simulink model "DIG_IF_test"  (R2021b)
settings: Solver=FixedStepDiscrete  StartTime=0.0  StopTime=stop_time-1  RelTol=1e-3
undefined symbols (not defined in the file): input_bus
libraries: dspsrcs4 x22
settings Model: DataTypeOverride=Off  Creator=torha  LastModifiedBy=torha
settings SolverCC: AlgebraicLoopSolver=TrustRegion
settings OptimizationCC: BlockReduction=off  ConditionallyExecuteInputs=off  DefaultParameterBehavior=Inlined  InheritOutputTypeSmallerThanSingle=on
settings DebuggingCC: AlgebraicLoopMsg=error  SingleTaskRateTransMsg=error  SFMachineParentedDataDiag=warning
settings HardwareCC: ProdBitPerPointer=32  ProdBitPerSizeT=32  ProdBitPerPtrDiffT=32  ProdLargestAtomicFloat=None  ProdIntDivRoundTo=Undefined  ProdEndianess=Unspecified  ProdWordSize=32  ProdHWDeviceType=ASIC/FPGA->ASIC/FPGA  TargetBitPerPointer=64  TargetBitPerSizeT=64  TargetBitPerPtrDiffT=64  TargetLongLongMode=on  TargetIntDivRoundTo=Zero  TargetEndianess=LittleEndian  TargetWordSize=64  TargetHWDeviceType=Custom Processor->MATLAB Host Computer  ProdEqTarget=off

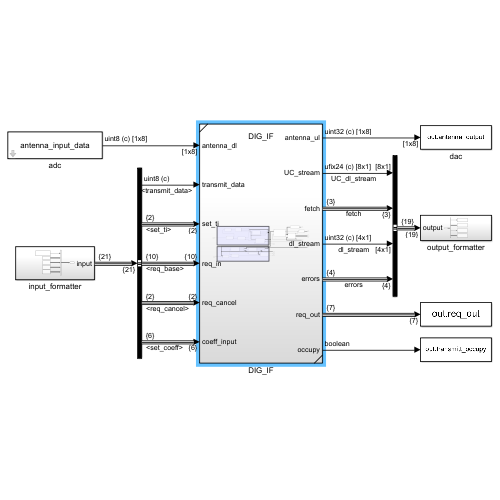
[thumbnail: Simulink's stored preview of the top-level diagram]
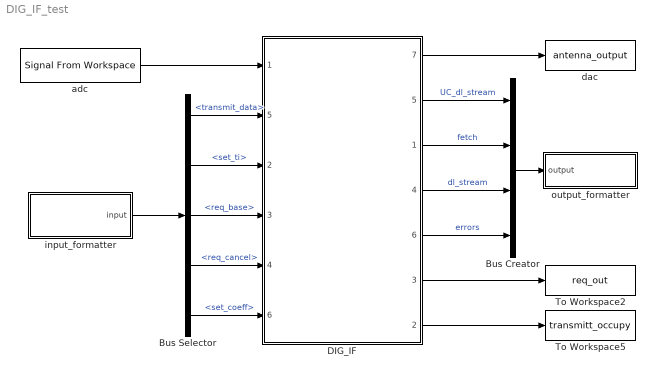
== system DIG_IF_test ==
  Bus Creator : BusCreator  Inputs=4
  Bus Selector : BusSelector  OutputSignals=transmit_data,set_ti,req_base,req_cancel,set_coeff
  DIG_IF : Subsystem  ReferencedSubsystem=DIG_IF
      settings: PortSchema="{\"entries\":[{\"content\":{\"sides\":[{\"content\":{\"connectorIds\":[\"Out7\",\"Out5\",\"Out1\",\"Out4\",\"Out6\",\"Out3\",\"Out2\"]},\"type\":\"ConnectorPlacement.EquallySpacedRectSide\",\"uuid\":\"0a36bb2c-b508-4463-a150-0627b474e72d\"},{\"content\":{\"connectorIds\":[\"In1\",\"In5\",\"In2\",\"In3\",\"In4\",\"In6\"],\"side\":\"RIGHT\"},\"type\":\"ConnectorPlacement.EquallySpacedRectSide\",\"uuid\":\"4cc461b4-d2d5-47e9-bf85-abb0cb83a1e3\"},{\"content\":{\"connectorIds\":[],\"side\":\"TOP\"},\"type\":\"ConnectorPlacement.EquallySpacedRectSide\",\"uuid\":\"3f3acd78-cd76-4a3f-93f8-4cd9f7c1daae\"},{\"content\":{\"connectorIds\":[],\"side\":\"BOTTOM\"},\"type\":\"ConnectorPlacement.EquallySpacedRectSide\",\"uuid\":\"e0439bc9-96cc-469d-b0c1-4082506a186c\"}]},\"type\":\"ConnectorPlacement.EquallySpacedConnector\",\"uuid\":\"66db1979-25ee-4b63-8861-56a9b0aa4b63\"}],\"packageUris\":[\"http://schema.mathworks.com/mf0/Connector/R2020b\"],\"version\":\"1.0\"}"
  To Workspace2 : ToWorkspace  VariableName=req_out  SaveFormat=Timeseries  SampleTime=-1
      settings: Save2DSignal=2-D array (concatenate along first dimension)
  To Workspace5 : ToWorkspace  VariableName=transmitt_occupy  SampleTime=-1
      settings: Save2DSignal=2-D array (concatenate along first dimension)
  adc : dspsrcs4/Signal From Workspace  X=antenna_input_data  Ts=1  nsamps=1  OutputAfterFinalValue=Setting to zero  ignoreOrWarnInputAndFrameLengths=off  OutputFrames=off
  dac : ToWorkspace  VariableName=antenna_output  SaveFormat=Timeseries  SampleTime=-1
  input_formatter : Subsystem
  output_formatter : Subsystem
  wires:
  Bus Selector/1 -> DIG_IF/5  "<transmit_data>"
  adc/1 -> DIG_IF/1
  DIG_IF/7 -> dac/1
  DIG_IF/2 -> To Workspace5/1
  DIG_IF/3 -> To Workspace2/1
  Bus Selector/3 -> DIG_IF/3  "<req_base>"
  Bus Selector/5 -> DIG_IF/6  "<set_coeff>"
  Bus Selector/2 -> DIG_IF/2  "<set_ti>"
  Bus Selector/4 -> DIG_IF/4  "<req_cancel>"
  input_formatter/1(input) -> Bus Selector/1
  DIG_IF/5 -> Bus Creator/1  "UC_dl_stream"
  DIG_IF/1 -> Bus Creator/2  "fetch"
  DIG_IF/4 -> Bus Creator/3  "dl_stream"
  DIG_IF/6 -> Bus Creator/4  "errors"
  Bus Creator/1 -> output_formatter/1(output)

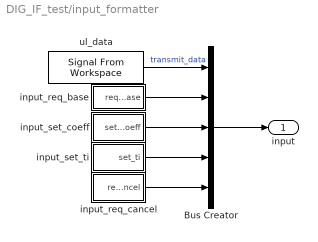
== system DIG_IF_test/input_formatter ==
  Bus Creator : BusCreator  Inputs=5
  input_req_base : Subsystem
  input_req_cancel : Subsystem
  input_set_coeff : Subsystem
  input_set_ti : Subsystem
  ul_data : dspsrcs4/Signal From Workspace  X=input_transmit_data  Ts=1  nsamps=1  OutputAfterFinalValue=Setting to zero  ignoreOrWarnInputAndFrameLengths=off  OutputFrames=off
  input : Outport
  wires:
  input_req_cancel/1(req_cancel) -> Bus Creator/5
  input_set_ti/1(set_ti) -> Bus Creator/4
  input_set_coeff/1(set_coeff) -> Bus Creator/3
  input_req_base/1(req_base) -> Bus Creator/2
  Bus Creator/1 -> input/1
  ul_data/1 -> Bus Creator/1  "transmit_data"

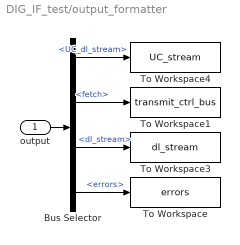
== system DIG_IF_test/output_formatter ==
  output : Inport
  Bus Selector : BusSelector  OutputSignals=UC_dl_stream,fetch,dl_stream,errors
  To Workspace : ToWorkspace  VariableName=errors  SaveFormat=Timeseries  SampleTime=-1
  To Workspace1 : ToWorkspace  VariableName=transmit_ctrl_bus  SaveFormat=Timeseries  SampleTime=-1
  To Workspace3 : ToWorkspace  VariableName=dl_stream  SampleTime=-1
      settings: Save2DSignal=2-D array (concatenate along first dimension)
  To Workspace4 : ToWorkspace  VariableName=UC_stream  SampleTime=-1
      settings: Save2DSignal=2-D array (concatenate along first dimension)
  wires:
  Bus Selector/3 -> To Workspace3/1  "<dl_stream>"
  Bus Selector/4 -> To Workspace/1  "<errors>"
  Bus Selector/1 -> To Workspace4/1  "<UC_dl_stream>"
  Bus Selector/2 -> To Workspace1/1  "<fetch>"
  output/1 -> Bus Selector/1

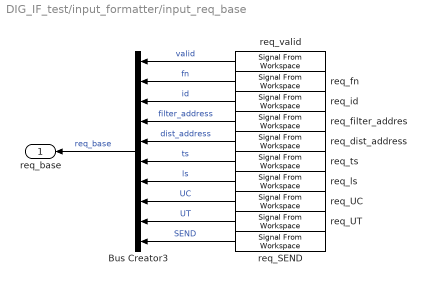
== system DIG_IF_test/input_formatter/input_req_base ==
  Bus Creator3 : BusCreator  Inputs=10
  req_SEND : dspsrcs4/Signal From Workspace  X=[horzcat([input_bus.req_base]).SEND].'  Ts=1  nsamps=1  OutputAfterFinalValue=Setting to zero  ignoreOrWarnInputAndFrameLengths=off  OutputFrames=off
  req_UC : dspsrcs4/Signal From Workspace  X=[horzcat([input_bus.req_base]).UC].'  Ts=1  nsamps=1  OutputAfterFinalValue=Setting to zero  ignoreOrWarnInputAndFrameLengths=off  OutputFrames=off
  req_UT : dspsrcs4/Signal From Workspace  X=[horzcat([input_bus.req_base]).UT].'  Ts=1  nsamps=1  OutputAfterFinalValue=Setting to zero  ignoreOrWarnInputAndFrameLengths=off  OutputFrames=off
  req_dist_address : dspsrcs4/Signal From Workspace  X=[horzcat([input_bus.req_base]).dist_address].'  Ts=1  nsamps=1  OutputAfterFinalValue=Setting to zero  ignoreOrWarnInputAndFrameLengths=off  OutputFrames=off
  req_filter_addres : dspsrcs4/Signal From Workspace  X=[horzcat([input_bus.req_base]).filter_address].'  Ts=1  nsamps=1  OutputAfterFinalValue=Setting to zero  ignoreOrWarnInputAndFrameLengths=off  OutputFrames=off
  req_fn : dspsrcs4/Signal From Workspace  X=[horzcat([input_bus.req_base]).fn].'  Ts=1  nsamps=1  OutputAfterFinalValue=Setting to zero  ignoreOrWarnInputAndFrameLengths=off  OutputFrames=off
  req_id : dspsrcs4/Signal From Workspace  X=[horzcat([input_bus.req_base]).id].'  Ts=1  nsamps=1  OutputAfterFinalValue=Setting to zero  ignoreOrWarnInputAndFrameLengths=off  OutputFrames=off
  req_ls : dspsrcs4/Signal From Workspace  X=[horzcat([input_bus.req_base]).ls].'  Ts=1  nsamps=1  OutputAfterFinalValue=Setting to zero  ignoreOrWarnInputAndFrameLengths=off  OutputFrames=off
  req_ts : dspsrcs4/Signal From Workspace  X=[horzcat([input_bus.req_base]).ts].'  Ts=1  nsamps=1  OutputAfterFinalValue=Setting to zero  ignoreOrWarnInputAndFrameLengths=off  OutputFrames=off
  req_valid : dspsrcs4/Signal From Workspace  X=[horzcat([input_bus.req_base]).valid].'  Ts=1  nsamps=1  OutputAfterFinalValue=Setting to zero  ignoreOrWarnInputAndFrameLengths=off  OutputFrames=off
  req_base : Outport
  wires:
  req_UC/1 -> Bus Creator3/8  "UC"
  req_filter_addres/1 -> Bus Creator3/4  "filter_address"
  req_dist_address/1 -> Bus Creator3/5  "dist_address"
  req_fn/1 -> Bus Creator3/2  "fn"
  req_UT/1 -> Bus Creator3/9  "UT"
  req_SEND/1 -> Bus Creator3/10  "SEND"
  req_valid/1 -> Bus Creator3/1  "valid"
  req_ls/1 -> Bus Creator3/7  "ls"
  req_id/1 -> Bus Creator3/3  "id"
  req_ts/1 -> Bus Creator3/6  "ts"
  Bus Creator3/1 -> req_base/1  "req_base"

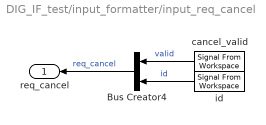
== system DIG_IF_test/input_formatter/input_req_cancel ==
  Bus Creator4 : BusCreator  Inputs=2
  cancel_valid : dspsrcs4/Signal From Workspace  X=[horzcat([input_bus.req_cancel]).valid].'  Ts=1  nsamps=1  OutputAfterFinalValue=Setting to zero  ignoreOrWarnInputAndFrameLengths=off  OutputFrames=off
  id : dspsrcs4/Signal From Workspace  X=[horzcat([input_bus.req_cancel]).id].'  Ts=1  nsamps=1  OutputAfterFinalValue=Setting to zero  ignoreOrWarnInputAndFrameLengths=off  OutputFrames=off
  req_cancel : Outport
  wires:
  id/1 -> Bus Creator4/2  "id"
  cancel_valid/1 -> Bus Creator4/1  "valid"
  Bus Creator4/1 -> req_cancel/1  "req_cancel"

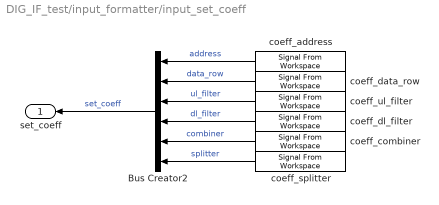
== system DIG_IF_test/input_formatter/input_set_coeff ==
  Bus Creator2 : BusCreator  Inputs=6
  coeff_address : dspsrcs4/Signal From Workspace  X=[horzcat([input_bus.set_coeff]).address].'  Ts=1  nsamps=1  OutputAfterFinalValue=Setting to zero  ignoreOrWarnInputAndFrameLengths=off  OutputFrames=off
  coeff_combiner : dspsrcs4/Signal From Workspace  X=[horzcat([input_bus.set_coeff]).combiner].'  Ts=1  nsamps=1  OutputAfterFinalValue=Setting to zero  ignoreOrWarnInputAndFrameLengths=off  OutputFrames=off
  coeff_data_row : dspsrcs4/Signal From Workspace  X=[horzcat([input_bus.set_coeff]).data_row].'  Ts=1  nsamps=1  OutputAfterFinalValue=Setting to zero  ignoreOrWarnInputAndFrameLengths=off  OutputFrames=off
  coeff_dl_filter : dspsrcs4/Signal From Workspace  X=[horzcat([input_bus.set_coeff]).dl_filter].'  Ts=1  nsamps=1  OutputAfterFinalValue=Setting to zero  ignoreOrWarnInputAndFrameLengths=off  OutputFrames=off
  coeff_splitter : dspsrcs4/Signal From Workspace  X=[horzcat([input_bus.set_coeff]).splitter].'  Ts=1  nsamps=1  OutputAfterFinalValue=Setting to zero  ignoreOrWarnInputAndFrameLengths=off  OutputFrames=off
  coeff_ul_filter : dspsrcs4/Signal From Workspace  X=[horzcat([input_bus.set_coeff]).ul_filter].'  Ts=1  nsamps=1  OutputAfterFinalValue=Setting to zero  ignoreOrWarnInputAndFrameLengths=off  OutputFrames=off
  set_coeff : Outport
  wires:
  coeff_ul_filter/1 -> Bus Creator2/3  "ul_filter"
  coeff_dl_filter/1 -> Bus Creator2/4  "dl_filter"
  coeff_address/1 -> Bus Creator2/1  "address"
  coeff_splitter/1 -> Bus Creator2/6  "splitter"
  coeff_data_row/1 -> Bus Creator2/2  "data_row"
  coeff_combiner/1 -> Bus Creator2/5  "combiner"
  Bus Creator2/1 -> set_coeff/1  "set_coeff"

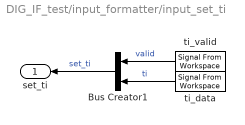
== system DIG_IF_test/input_formatter/input_set_ti ==
  Bus Creator1 : BusCreator  Inputs=2
  ti_data : dspsrcs4/Signal From Workspace  X=[horzcat([input_bus.set_ti]).ti].'  Ts=1  nsamps=1  OutputAfterFinalValue=Setting to zero  ignoreOrWarnInputAndFrameLengths=off  OutputFrames=off
  ti_valid : dspsrcs4/Signal From Workspace  X=[horzcat([input_bus.set_ti]).valid].'  Ts=1  nsamps=1  OutputAfterFinalValue=Setting to zero  ignoreOrWarnInputAndFrameLengths=off  OutputFrames=off
  set_ti : Outport
  wires:
  ti_valid/1 -> Bus Creator1/1  "valid"
  ti_data/1 -> Bus Creator1/2  "ti"
  Bus Creator1/1 -> set_ti/1  "set_ti"
